simulink model "CircularTrajectory"  (R2017b)
settings: Solver=ode4  StartTime=0.0  StopTime=tsim  FixedStep=baseRate  RelTol=1e-3  EnableMultiTasking=on
values from neighbouring files (symbols this model uses):
  drop_states_BLACK = [1.36947387695313,1.22175756835938,-0.0161599479615688]    [Run_Initializer.m]
  drop_states_RED = [2.18401342773438,1.21458435058594,-3.12528014183044]    [Run_Initializer.m]
  home_states_BLACK = [ xLength/2; yLength/2; 0]    [Run_Initializer.m]
  home_states_RED = [ xLength/2+0.7; yLength/2; pi]    [Run_Initializer.m]
  init_states_BLACK = [ xLength/2; yLength/2; 0]    [Run_Initializer.m]
  init_states_RED = [ xLength/2+0.7; yLength/2; pi]    [Run_Initializer.m]
  Kd_tb = 0.4    [Run_Initializer.m]
  Kd_tr = 0.4    [Run_Initializer.m]
  Kd_xb = 5    [Run_Initializer.m]
  Kd_xr = 5    [Run_Initializer.m]
  Kd_yb = 5    [Run_Initializer.m]
  Kd_yr = 5    [Run_Initializer.m]
  Kp_tb = 0.1    [Run_Initializer.m]
  Kp_tr = 0.1    [Run_Initializer.m]
  Kp_xb = 2    [Run_Initializer.m]
  Kp_xr = 2    [Run_Initializer.m]
  Kp_yb = 2    [Run_Initializer.m]
  Kp_yr = 2    [Run_Initializer.m]
  noise_variance_BLACK = 0    [Run_Initializer.m]
  noise_variance_RED = 0    [Run_Initializer.m]
  Phase0_End = Phase0_Duration    (= 10)    [Run_Initializer.m]
  Phase1_End = Phase0_Duration + Phase1_Duration    (= 15)    [Run_Initializer.m]
  Phase2_End = Phase0_Duration + Phase1_Duration +                                   Phase2_Duration    (= 35)    [Run_Initializer.m]
  Phase3_End = Phase0_Duration + Phase1_Duration +                                   Phase2_Duration + Phase3_Duration    (= 166)    [Run_Initializer.m]
  Phase3_SubPhase1_End = Phase2_End + Phase3_SubPhase1_Duration    (= 40)    [Run_Initializer.m]
  Phase3_SubPhase2_End = Phase2_End + Phase3_SubPhase1_Duration +                                   Phase3_SubPhase2_Duration    (= 45)    [Run_Initializer.m]
  Phase3_SubPhase3_End = Phase2_End + Phase3_SubPhase1_Duration +                                   Phase3_SubPhase2_Duration +                                  Phase3_SubPhase3_Duration    (= 46)    [Run_Initializer.m]
  Phase3_SubPhase4_End = Phase2_End + Phase3_SubPhase1_Duration +                                   Phase3_SubPhase2_Duration +                                  Phase3_SubPhase3_Duration +                                  Phase3_SubPhase4_Duration    [Run_Initializer.m]
  Phase4_End = Phase0_Duration + Phase1_Duration +                                   Phase2_Duration + Phase3_Duration +                                   Phase4_Duration    (= 186)    [Run_Initializer.m]
  Phase5_End = Phase0_Duration + Phase1_Duration +                                   Phase2_Duration + Phase3_Duration +                                   Phase4_Duration + Phase5_Duration    (= 191)    [Run_Initializer.m]
  serverRate = 0.1    [Run_Initializer.m]
  xLength = 3.51155    [Run_Initializer.m]
  yLength = 2.41935    [Run_Initializer.m]
undefined symbols (not defined in the file or in its folder): DiscIntNeverNeededParam, F_thrusters_BLACK, F_thrusters_RED, platformSelection, simMode, thruster_dist2CG_BLACK, thruster_dist2CG_RED
libraries: MainLibrary x22, GPIOLibrary x20, raspberrypilib x17, embdlinuxlib x6, dspsigops x5, dspswit3 x2
(part 5 of 5)

== system CircularTrajectory/Phase #3: Experiment/Change RED Behavior/Sub-Phase #1/Custom Discrete PD (X-Position)/x_dot -> x1/Hold this value ==
  In1 : Inport
  Action Port : ActionPort  ActionType=then
  Out1 : Outport
  wires:
  In1/1 -> Out1/1

== system CircularTrajectory/Phase #3: Experiment/Change RED Behavior/Sub-Phase #1/Custom Discrete PD (Y-Position)/x_dot -> x1/Hold this value ==
  In1 : Inport
  Action Port : ActionPort  ActionType=then
  Out1 : Outport
  wires:
  In1/1 -> Out1/1

== system CircularTrajectory/Phase #3: Experiment/Change RED Behavior/Sub-Phase #4/Custom Discrete PD (Attitude)/x_dot -> x1/Hold this value ==
  In1 : Inport
  Action Port : ActionPort  ActionType=then
  Out1 : Outport
  wires:
  In1/1 -> Out1/1

== system CircularTrajectory/Phase #3: Experiment/Change RED Behavior/Sub-Phase #4/Custom Discrete PD (X-Position)/x_dot -> x1/Hold this value ==
  In1 : Inport
  Action Port : ActionPort  ActionType=then
  Out1 : Outport
  wires:
  In1/1 -> Out1/1

== system CircularTrajectory/Phase #3: Experiment/Change RED Behavior/Sub-Phase #4/Custom Discrete PD (Y-Position)/x_dot -> x1/Hold this value ==
  In1 : Inport
  Action Port : ActionPort  ActionType=then
  Out1 : Outport
  wires:
  In1/1 -> Out1/1

== matlab function CircularTrajectory/Phase #3: Experiment/Change BLACK Behavior/Sub-Phase #4/BLACK_RzD/Wrap1/MATLAB Function ==
  data: u input; wrappedAngle output
function wrappedAngle = wrapAngle(u)

wrappedAngle = atan2(sin(u),cos(u));

end

== matlab function CircularTrajectory/Simulate Plant Dynamics/RED Dynamics Model/MATLAB Function ==
  data: control_inputs input; x_ddot output; model_param parameter
function x_ddot = RED_dynamics(control_inputs, model_param)

%#codegen
% Fully define the size of x_ddot() for code generation:
x_ddot     = zeros(3,1);

% Extract the servicer model parameters from the model_param vector defined
% in initialize.m:
m_RED    = model_param(1);
I_RED    = model_param(2);

% Extract the control inputs from the control_input vector:
Fx        = control_inputs(1);              % [N]
Fy        = control_inputs(2);              % [N]
Tz        = control_inputs(3);              % [N.m]

% Calculate the state acceleration vector:
x_ddot(1) = Fx/m_RED;                      % [m/s^2]
x_ddot(2) = Fy/m_RED;                      % [m/s^2]
x_ddot(3) = Tz/I_RED;                      % [rad/s^2]

end

== matlab function CircularTrajectory/Simulate Plant Dynamics/BLACK Dynamics Model/MATLAB Function ==
  data: control_inputs input; x_ddot output; model_param parameter
function x_ddot = BLACK_dynamics(control_inputs, model_param)

%#codegen
% Fully define the size of x_ddot() for code generation:
x_ddot     = zeros(3,1);

% Extract the servicer model parameters from the model_param vector defined
% in initialize.m:
m_BLACK    = model_param(3);
I_BLACK    = model_param(4);

% Extract the control inputs from the control_input vector:
Fx        = control_inputs(1);              % [N]
Fy        = control_inputs(2);              % [N]
Tz        = control_inputs(3);              % [N.m]

% Calculate the state acceleration vector:
x_ddot(1) = Fx/m_BLACK;                      % [m/s^2]
x_ddot(2) = Fy/m_BLACK;                      % [m/s^2]
x_ddot(3) = Tz/I_BLACK;                      % [rad/s^2]

end

== matlab function CircularTrajectory/Phase #4: Return Home/Change BLACK Behavior/Hough Control/MATLAB Function2 ==
  data: Oy output; z input; Ox output
function [Oy, Ox]   = C3( z )
%C3 gives the rotation matrix about the z-axis for an angle 'z'
%   z - the angle about the z-axis which you rotate
%   A - the rotation matrix

Ox = [cos(z) sin(z); -sin(z) cos(z)]*[1;0];
Oy = [cos(z) sin(z); -sin(z) cos(z)]*[0;1];
end

== matlab function CircularTrajectory/From Force//Torque, Command Thrusters/Change RED Behavior/Rotate Forces to Body/Create Rotation Matrix ==
  data: Rz input; C_bI output
function C_bI = RotateFrame(Rz)

C_bI = [  cos(Rz) sin(Rz)
         -sin(Rz) cos(Rz) ];

end

== matlab function CircularTrajectory/From Force//Torque, Command Thrusters/Change BLACK Behavior/Calculate Thruster ON//OFF/MATLAB Function ==
  data: H output; thruster_dist2CG_BLACK parameter; F_thrusters_BLACK parameter
function H = MakeH(thruster_dist2CG_BLACK,F_thrusters_BLACK)

Vec1 = [ -1
         -1
          0 
          0
          1
          1
          0
          0 ];
      
Vec2 = [  0
          0
          1
          1
          0
          0
         -1
         -1 ];
     
Vec3 = thruster_dist2CG_BLACK./1000;

Mat1 = [Vec1, Vec2, Vec3]';

Mat2 = diag((F_thrusters_BLACK./2));

H    = Mat1*Mat2;

end

== matlab function CircularTrajectory/From Force//Torque, Command Thrusters/Change RED Behavior/Calculate Thruster ON//OFF/MATLAB Function ==
  data: H output; thruster_dist2CG_RED parameter; F_thrusters_RED parameter
function H = MakeH(thruster_dist2CG_RED,F_thrusters_RED)

Vec1 = [ -1
         -1
          0 
          0
          1
          1
          0
          0 ];
      
Vec2 = [  0
          0
          1
          1
          0
          0
         -1
         -1 ];
     
Vec3 = thruster_dist2CG_RED./1000;

Mat1 = [Vec1, Vec2, Vec3]';

Mat2 = diag((F_thrusters_RED./2));

H    = Mat1*Mat2;

end

== matlab function CircularTrajectory/From Force//Torque, Command Thrusters/Change RED Behavior/Calculate Thruster ON//OFF/MATLAB Function1 ==
  data: H output; thruster_dist2CG_RED parameter; F_thrusters_RED parameter
function H = MakeH(thruster_dist2CG_RED,F_thrusters_RED)

Vec1 = [ -1
         -1
          0 
          0
          1
          1
          0
          0 ];
      
Vec2 = [  0
          0
          1
          1
          0
          0
         -1
         -1 ];
     
Vec3 = thruster_dist2CG_RED./1000;

Mat1 = [Vec1, Vec2, Vec3]';

Mat2 = diag((F_thrusters_RED));

H    = Mat1*Mat2;

end

== matlab function CircularTrajectory/From Force//Torque, Command Thrusters/Change RED Behavior/Calculate Thruster ON//OFF/MATLAB Function2 ==
  data: ThrustPer_Final output; ThrustPer input
function ThrustPer_Final  = ThrusterSat(ThrustPer)

ValveTime       = 0.007;
TControl        = 0.1;
ThrustPer_Final = zeros(8,1);

if max(ThrustPer) > 1
    ThrustPer_Sat = ThrustPer/max(ThrustPer);
else
    ThrustPer_Sat = ThrustPer;
end

for i = 1:8
    if ThrustPer_Sat(i) > ValveTime/TControl 
        ThrustPer_Final(i) = ThrustPer_Sat(i);
    else
        ThrustPer_Final(i) = 0;
    end
end
   

end

== matlab function CircularTrajectory/From Force//Torque, Command Thrusters/Change RED Behavior/Calculate Thruster ON//OFF/Rotate Forces to Inertial/Create Rotation Matrix ==
  data: Rz input; C_Ib output
function C_Ib = RotateFrame(Rz)

C_bI = [  cos(Rz) sin(Rz)
         -sin(Rz) cos(Rz) ];

C_Ib = inv(C_bI);

end

== matlab function CircularTrajectory/From Force//Torque, Command Thrusters/Change BLACK Behavior/Calculate Thruster ON//OFF/MATLAB Function1 ==
  data: H output; thruster_dist2CG_BLACK parameter; F_thrusters_BLACK parameter
function H = MakeH(thruster_dist2CG_BLACK,F_thrusters_BLACK)

Vec1 = [ -1
         -1
          0 
          0
          1
          1
          0
          0 ];
      
Vec2 = [  0
          0
          1
          1
          0
          0
         -1
         -1 ];
     
Vec3 = thruster_dist2CG_BLACK./1000;

Mat1 = [Vec1, Vec2, Vec3]';

Mat2 = diag((F_thrusters_BLACK));

H    = Mat1*Mat2;

end

== matlab function CircularTrajectory/From Force//Torque, Command Thrusters/Change BLACK Behavior/Calculate Thruster ON//OFF/MATLAB Function2 ==
  data: ThrustPer_Final output; ThrustPer input
function ThrustPer_Final  = ThrusterSat(ThrustPer)

ValveTime       = 0.007;
TControl        = 0.1;
ThrustPer_Final = zeros(8,1);

if max(ThrustPer) > 1
    ThrustPer_Sat = ThrustPer/max(ThrustPer);
else
    ThrustPer_Sat = ThrustPer;
end

for i = 1:8
    if ThrustPer_Sat(i) > ValveTime/TControl 
        ThrustPer_Final(i) = ThrustPer_Sat(i);
    else
        ThrustPer_Final(i) = 0;
    end
end
   

end

== matlab function CircularTrajectory/Phase #2: Move to Initial Position/Change BLACK Behavior/Hough Control/MATLAB Function2 ==
  data: Oy output; z input; Ox output
function [Oy, Ox]   = C3( z )
%C3 gives the rotation matrix about the z-axis for an angle 'z'
%   z - the angle about the z-axis which you rotate
%   A - the rotation matrix

Ox = [cos(z) sin(z); -sin(z) cos(z)]*[1;0];
Oy = [cos(z) sin(z); -sin(z) cos(z)]*[0;1];
end

== matlab function CircularTrajectory/From Force//Torque, Command Thrusters/Change BLACK Behavior/Calculate Thruster ON//OFF/Rotate Forces to Inertial/Create Rotation Matrix ==
  data: Rz input; C_Ib output
function C_Ib = RotateFrame(Rz)

C_bI = [  cos(Rz) sin(Rz)
         -sin(Rz) cos(Rz) ];

C_Ib = inv(C_bI);

end

== matlab function CircularTrajectory/From Force//Torque, Command Thrusters/Change BLACK Behavior/Rotate Forces to Body/Create Rotation Matrix ==
  data: Rz input; C_bI output
function C_bI = RotateFrame(Rz)

C_bI = [  cos(Rz) sin(Rz)
         -sin(Rz) cos(Rz) ];

end

== matlab function CircularTrajectory/From Torque, Command RW/Change RED Behavior/Calculate Saturated RPM Signal/Calculate RW RPM Increment ==
  data: Tz_Sat input; dRPM_RW output; baseRate parameter
function dRPM_RW = Calc_RW_RPM(Tz_Sat,baseRate)

dRPM_RW =  (Tz_Sat/0.007244720)*(60/2/pi)*baseRate;

end

== matlab function CircularTrajectory/From Torque, Command RW/Change RED Behavior/Wheel RPM to PWM/Check if RW is Ready ==
  data: Status input; EnableSig output; WheelRPM_In input; WheelRPM_Out output
function [EnableSig, WheelRPM_Out] = Check_Wheel_Status(Status, WheelRPM_In)

if Status == 0
    EnableSig    = 1;
    WheelRPM_Out = WheelRPM_In;
else
    EnableSig    = 0;
    WheelRPM_Out = 0;
end

end

== matlab function CircularTrajectory/Phase #2: Move to Initial Position/Change BLACK Behavior/Hough Control/MATLAB Function3 ==
  data: z input; Ox output
function Ox    = C3( z )
%C3 gives the rotation matrix about the z-axis for an angle 'z'
%   z - the angle about the z-axis which you rotate
%   A - the rotation matrix

Ox = [cos(z) sin(z); -sin(z) cos(z)]*[1;0];
end

== matlab function CircularTrajectory/From Torque, Command RW/Change RED Behavior/Wheel RPM to PWM/RPM to PWM Value ==
  data: MotorRPM_Sat input; WheelPWM output
function WheelPWM = RPM2PWM(MotorRPM_Sat)

PWMRange = 0.9-0.1;

WheelPWM = ((MotorRPM_Sat*PWMRange)/7000) + 0.1;

end

== matlab function CircularTrajectory/From Torque, Command RW/Change RED Behavior/Wheel RPM to PWM/Get RW Direction ==
  data: MotorRPM_Sat input; WheelDirection output
function WheelDirection = GetDirection(MotorRPM_Sat)

if MotorRPM_Sat > 0
    WheelDirection = 0;
else
    WheelDirection = 1;
end
        
end

== matlab function CircularTrajectory/Phase #3: Experiment/Change BLACK Behavior/Sub-Phase #4/Hough Control/MATLAB Function2 ==
  data: Oy output; z input; Ox output
function [Oy, Ox]   = C3( z )
%C3 gives the rotation matrix about the z-axis for an angle 'z'
%   z - the angle about the z-axis which you rotate
%   A - the rotation matrix

Ox = [cos(z) sin(z); -sin(z) cos(z)]*[1;0];
Oy = [cos(z) sin(z); -sin(z) cos(z)]*[0;1];
end

== matlab function CircularTrajectory/Phase #2: Move to Initial Position/Change BLACK Behavior/Hough Control/MATLAB Function4 ==
  data: Oy input; e_out output; e_in input
function e_out = fcn(Oy, e_in)

a = sign(Oy'*e_in);
e_out = -a*norm(e_in);

== matlab function CircularTrajectory/Phase #3: Experiment/Change BLACK Behavior/Sub-Phase #4/Hough Control/MATLAB Function3 ==
  data: z input; Ox output
function Ox    = C3( z )
%C3 gives the rotation matrix about the z-axis for an angle 'z'
%   z - the angle about the z-axis which you rotate
%   A - the rotation matrix

Ox = [cos(z) sin(z); -sin(z) cos(z)]*[1;0];
end

== matlab function CircularTrajectory/Simulate Plant Dynamics/Sample and Hold Data to Match PhaseSpace (RED)/MATLAB Function ==
  data: TIME input; y output; SERVER input
function y = fcn(TIME, SERVER)

if mod(TIME,SERVER) == 0
    y = 1;
else
    y = 0;
end

== matlab function CircularTrajectory/Simulate Plant Dynamics/Sample and Hold Data to Match PhaseSpace (BLACK)/MATLAB Function ==
  data: TIME input; y output; SERVER input
function y = fcn(TIME, SERVER)

if mod(TIME,SERVER) == 0
    y = 1;
else
    y = 0;
end

== matlab function CircularTrajectory/Phase #4: Return Home/Change RED Behavior/Hough Control/MATLAB Function2 ==
  data: Oy output; z input; Ox output
function [Oy, Ox]   = C3( z )
%C3 gives the rotation matrix about the z-axis for an angle 'z'
%   z - the angle about the z-axis which you rotate
%   A - the rotation matrix

Ox = [cos(z) sin(z); -sin(z) cos(z)]*[1;0];
Oy = [cos(z) sin(z); -sin(z) cos(z)]*[0;1];
end

== matlab function CircularTrajectory/Phase #2: Move to Initial Position/Change RED Behavior/Hough Control/MATLAB Function2 ==
  data: Oy output; z input; Ox output
function [Oy, Ox]   = C3( z )
%C3 gives the rotation matrix about the z-axis for an angle 'z'
%   z - the angle about the z-axis which you rotate
%   A - the rotation matrix

Ox = [cos(z) sin(z); -sin(z) cos(z)]*[1;0];
Oy = [cos(z) sin(z); -sin(z) cos(z)]*[0;1];
end

== matlab function CircularTrajectory/Phase #2: Move to Initial Position/Change RED Behavior/Hough Control/MATLAB Function3 ==
  data: z input; Ox output
function Ox    = C3( z )
%C3 gives the rotation matrix about the z-axis for an angle 'z'
%   z - the angle about the z-axis which you rotate
%   A - the rotation matrix

Ox = [cos(z) sin(z); -sin(z) cos(z)]*[1;0];
end

== matlab function CircularTrajectory/Phase #2: Move to Initial Position/Change RED Behavior/Hough Control/MATLAB Function4 ==
  data: Oy input; e_out output; e_in input
function e_out = fcn(Oy, e_in)

a = sign(Oy'*e_in);
e_out = -a*norm(e_in);

== matlab function CircularTrajectory/Phase #4: Return Home/Change RED Behavior/Hough Control/MATLAB Function3 ==
  data: z input; Ox output
function Ox    = C3( z )
%C3 gives the rotation matrix about the z-axis for an angle 'z'
%   z - the angle about the z-axis which you rotate
%   A - the rotation matrix

Ox = [cos(z) sin(z); -sin(z) cos(z)]*[1;0];
end

== matlab function CircularTrajectory/Phase #4: Return Home/Change RED Behavior/Hough Control/MATLAB Function4 ==
  data: Oy input; e_out output; e_in input
function e_out = fcn(Oy, e_in)

a = sign(Oy'*e_in);
e_out = -a*norm(e_in);

== matlab function CircularTrajectory/Phase #4: Return Home/Change BLACK Behavior/Hough Control/MATLAB Function3 ==
  data: z input; Ox output
function Ox    = C3( z )
%C3 gives the rotation matrix about the z-axis for an angle 'z'
%   z - the angle about the z-axis which you rotate
%   A - the rotation matrix

Ox = [cos(z) sin(z); -sin(z) cos(z)]*[1;0];
end

== matlab function CircularTrajectory/Phase #4: Return Home/Change BLACK Behavior/Hough Control/MATLAB Function4 ==
  data: Oy input; e_out output; e_in input
function e_out = fcn(Oy, e_in)

a = sign(Oy'*e_in);
e_out = -a*norm(e_in);

== matlab function CircularTrajectory/Phase #3: Experiment/Change RED Behavior/Sub-Phase #1/Hough Control/MATLAB Function2 ==
  data: Oy output; z input; Ox output
function [Oy, Ox]   = C3( z )
%C3 gives the rotation matrix about the z-axis for an angle 'z'
%   z - the angle about the z-axis which you rotate
%   A - the rotation matrix

Ox = [cos(z) sin(z); -sin(z) cos(z)]*[1;0];
Oy = [cos(z) sin(z); -sin(z) cos(z)]*[0;1];
end

== matlab function CircularTrajectory/Phase #3: Experiment/Change RED Behavior/Sub-Phase #1/Hough Control/MATLAB Function3 ==
  data: z input; Ox output
function Ox    = C3( z )
%C3 gives the rotation matrix about the z-axis for an angle 'z'
%   z - the angle about the z-axis which you rotate
%   A - the rotation matrix

Ox = [cos(z) sin(z); -sin(z) cos(z)]*[1;0];
end

== matlab function CircularTrajectory/Phase #3: Experiment/Change RED Behavior/Sub-Phase #1/Hough Control/MATLAB Function4 ==
  data: Oy input; e_out output; e_in input
function e_out = fcn(Oy, e_in)

a = sign(Oy'*e_in);
e_out = -a*norm(e_in);

== matlab function CircularTrajectory/Phase #3: Experiment/Change RED Behavior/Sub-Phase #4/Hough Control/MATLAB Function2 ==
  data: Oy output; z input; Ox output
function [Oy, Ox]   = C3( z )
%C3 gives the rotation matrix about the z-axis for an angle 'z'
%   z - the angle about the z-axis which you rotate
%   A - the rotation matrix

Ox = [cos(z) sin(z); -sin(z) cos(z)]*[1;0];
Oy = [cos(z) sin(z); -sin(z) cos(z)]*[0;1];
end

== matlab function CircularTrajectory/Phase #3: Experiment/Change RED Behavior/Sub-Phase #4/Hough Control/MATLAB Function3 ==
  data: z input; Ox output
function Ox    = C3( z )
%C3 gives the rotation matrix about the z-axis for an angle 'z'
%   z - the angle about the z-axis which you rotate
%   A - the rotation matrix

Ox = [cos(z) sin(z); -sin(z) cos(z)]*[1;0];
end

== matlab function CircularTrajectory/Phase #3: Experiment/Change RED Behavior/Sub-Phase #4/Hough Control/MATLAB Function4 ==
  data: Oy input; e_out output; e_in input
function e_out = fcn(Oy, e_in)

a = sign(Oy'*e_in);
e_out = -a*norm(e_in);

== matlab function CircularTrajectory/Phase #3: Experiment/Change BLACK Behavior/Sub-Phase #4/Hough Control/MATLAB Function4 ==
  data: Oy input; e_out output; e_in input
function e_out = fcn(Oy, e_in)

a = sign(Oy'*e_in);
e_out = -a*norm(e_in);

== matlab function CircularTrajectory/Phase #3: Experiment/Change BLACK Behavior/Sub-Phase #1/Hough Control/MATLAB Function2 ==
  data: Oy output; z input; Ox output
function [Oy, Ox]   = C3( z )
%C3 gives the rotation matrix about the z-axis for an angle 'z'
%   z - the angle about the z-axis which you rotate
%   A - the rotation matrix

Ox = [cos(z) sin(z); -sin(z) cos(z)]*[1;0];
Oy = [cos(z) sin(z); -sin(z) cos(z)]*[0;1];
end

== matlab function CircularTrajectory/Phase #3: Experiment/Change BLACK Behavior/Sub-Phase #1/Hough Control/MATLAB Function3 ==
  data: z input; Ox output
function Ox    = C3( z )
%C3 gives the rotation matrix about the z-axis for an angle 'z'
%   z - the angle about the z-axis which you rotate
%   A - the rotation matrix

Ox = [cos(z) sin(z); -sin(z) cos(z)]*[1;0];
end

== matlab function CircularTrajectory/Phase #3: Experiment/Change BLACK Behavior/Sub-Phase #1/Hough Control/MATLAB Function4 ==
  data: Oy input; e_out output; e_in input
function e_out = fcn(Oy, e_in)

a = sign(Oy'*e_in);
e_out = -a*norm(e_in);

== matlab function CircularTrajectory/Phase #5: Hold Home/Change BLACK Behavior/Hough Control/MATLAB Function2 ==
  data: Oy output; z input; Ox output
function [Oy, Ox]   = C3( z )
%C3 gives the rotation matrix about the z-axis for an angle 'z'
%   z - the angle about the z-axis which you rotate
%   A - the rotation matrix

Ox = [cos(z) sin(z); -sin(z) cos(z)]*[1;0];
Oy = [cos(z) sin(z); -sin(z) cos(z)]*[0;1];
end

== matlab function CircularTrajectory/Phase #5: Hold Home/Change BLACK Behavior/Hough Control/MATLAB Function3 ==
  data: z input; Ox output
function Ox    = C3( z )
%C3 gives the rotation matrix about the z-axis for an angle 'z'
%   z - the angle about the z-axis which you rotate
%   A - the rotation matrix

Ox = [cos(z) sin(z); -sin(z) cos(z)]*[1;0];
end

== matlab function CircularTrajectory/Phase #5: Hold Home/Change BLACK Behavior/Hough Control/MATLAB Function4 ==
  data: Oy input; e_out output; e_in input
function e_out = fcn(Oy, e_in)

a = sign(Oy'*e_in);
e_out = -a*norm(e_in);

== matlab function CircularTrajectory/Calculate RED_Rz_Shoulder/Wrap2Pi ==
  data: angle_rad input; angle_rad_wrapped output
function angle_rad_wrapped = wrap2pi(angle_rad)

angle_rad_wrapped = angle_rad - 2*pi*floor( (angle_rad+pi)/(2*pi) ); 

end

== matlab function CircularTrajectory/Calculate RED_Rz_Elbow/Wrap2Pi1 ==
  data: angle_rad input; angle_rad_wrapped output
function angle_rad_wrapped = wrap2pi(angle_rad)

angle_rad_wrapped = angle_rad - 2*pi*floor( (angle_rad+pi)/(2*pi) ); 

end

== matlab function CircularTrajectory/Phase #5: Hold Home/Change RED Behavior/Hough Control/MATLAB Function2 ==
  data: Oy output; z input; Ox output
function [Oy, Ox]   = C3( z )
%C3 gives the rotation matrix about the z-axis for an angle 'z'
%   z - the angle about the z-axis which you rotate
%   A - the rotation matrix

Ox = [cos(z) sin(z); -sin(z) cos(z)]*[1;0];
Oy = [cos(z) sin(z); -sin(z) cos(z)]*[0;1];
end

== matlab function CircularTrajectory/Phase #5: Hold Home/Change RED Behavior/Hough Control/MATLAB Function3 ==
  data: z input; Ox output
function Ox    = C3( z )
%C3 gives the rotation matrix about the z-axis for an angle 'z'
%   z - the angle about the z-axis which you rotate
%   A - the rotation matrix

Ox = [cos(z) sin(z); -sin(z) cos(z)]*[1;0];
end

== matlab function CircularTrajectory/Phase #5: Hold Home/Change RED Behavior/Hough Control/MATLAB Function4 ==
  data: Oy input; e_out output; e_in input
function e_out = fcn(Oy, e_in)

a = sign(Oy'*e_in);
e_out = -a*norm(e_in);

== matlab function CircularTrajectory/Calculate RED_Rz_Wrist/Wrap2Pi2 ==
  data: angle_rad input; angle_rad_wrapped output
function angle_rad_wrapped = wrap2pi(angle_rad)

angle_rad_wrapped = angle_rad - 2*pi*floor( (angle_rad+pi)/(2*pi) ); 

end

== matlab function CircularTrajectory/Phase #3: Experiment/Change RED Behavior/Sub-Phase #4/MATLAB Function ==
  data: t input; x output; xLength parameter
function x = fcn(t, xLength)

x = 0.7*cos((0.104719755/2)*t) + xLength/2;

end

== matlab function CircularTrajectory/Phase #3: Experiment/Change RED Behavior/Sub-Phase #4/MATLAB Function1 ==
  data: t input; y output; yLength parameter
function y = fcn(t, yLength)

y = 0.7*sin((0.104719755/2)*t) + yLength/2;

end
